simulink model "E13_implementation"  (R2017a)
settings: Solver=VariableStepAuto  StartTime=0.0  StopTime=50  RelTol=1e-3
InitFcn:
  | clear
  | E_param
undefined symbols (not defined in the file or in its folder): E_animation
settings Model: Creator=Mat Haskell  LastModifiedBy=Mat Haskell

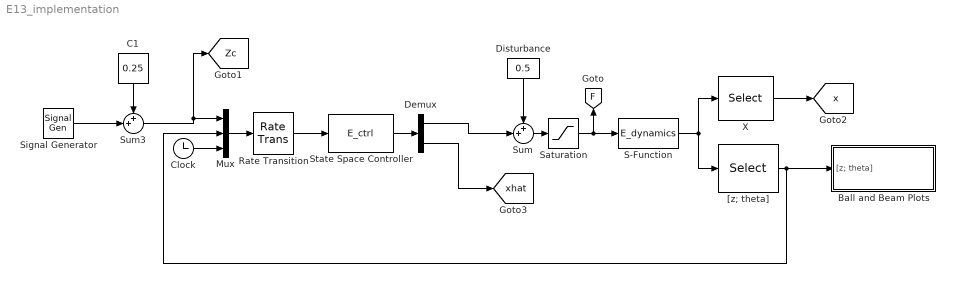
== system E13_implementation ==
  Ball and Beam Plots : Subsystem
  C1 : Constant  Value=0.25
  Clock : Clock
  Demux : Demux  Outputs=2
  Disturbance : Constant  Value=0.5
  Mux : Mux  Inputs=3
  Rate Transition : RateTransition  OutPortSampleTime=P.Ts
  S-Function : S-Function  FunctionName=E_dynamics  Parameters=P  SFunctionDeploymentMode=off  EnableBusSupport=off
  Saturation : Saturate  UpperLimit=15  LowerLimit=-15
  Signal Generator : SignalGenerator  WaveForm=square  Amplitude=.125  Frequency=.05
  State Space Controller : MATLABFcn  InitFcn=E_param  MATLABFcn=E_ctrl  OutputDimensions=5
  Sum : Sum  Inputs=++|
  Sum3 : Sum  Inputs=++|
  X : Selector  InputPortWidth=6  IndexOptions=Index vector (dialog)  Indices=[3 4 5 6]  OutputSizes=1
  "[z; theta]" : Selector  InputPortWidth=6  IndexOptions=Index vector (dialog)  Indices=[1 2]  OutputSizes=1
  tag scope: F=global, Zc=global, x=global, xhat=global
  wires:
  Sum3/1 -> [Zc], Mux/1
  Saturation/1 -> S-Function/1, [F]
  C1/1 -> Sum3/1
  Signal Generator/1 -> Sum3/2
  Sum/1 -> Saturation/1
  Disturbance/1 -> Sum/1
  Clock/1 -> Mux/3
  S-Function/1 -> X/1, "[z; theta]"/1
  X/1 -> [x]
  Demux/2 -> [xhat]
  "[z; theta]"/1 -> Mux/2, Ball and Beam Plots/1("[z; theta]")
  State Space Controller/1 -> Demux/1
  Demux/1 -> Sum/2
  Mux/1 -> Rate Transition/1
  Rate Transition/1 -> State Space Controller/1

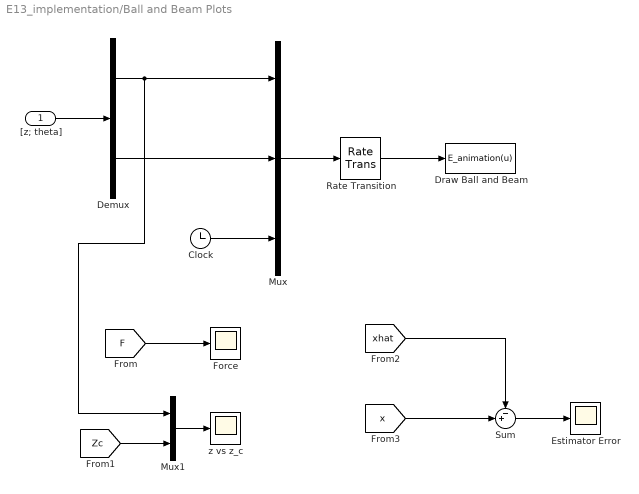
== system E13_implementation/Ball and Beam Plots ==
  "[z; theta]" : Inport
  Clock : Clock
  Demux : Demux  Outputs=2
  Draw Ball and Beam : MATLABFcn  MATLABFcn=E_animation(u)  OutputDimensions=0
  Estimator Error : Scope
  Force : Scope
  Mux : Mux  Inputs=3
  Mux1 : Mux  Inputs=2
  Rate Transition : RateTransition  OutPortSampleTime=P.t_plot
  Sum : Sum  Inputs=-+|
  z vs z_c : Scope
  wires:
  "[z; theta]"/1 -> Demux/1
  Rate Transition/1 -> Draw Ball and Beam/1
  Mux/1 -> Rate Transition/1
  Clock/1 -> Mux/3
  Demux/1 -> Mux1/1, Mux/1
  Demux/2 -> Mux/2
  [F] -> Force/1
  Mux1/1 -> z vs z_c/1
  [Zc] -> Mux1/2
  [xhat] -> Sum/1
  [x] -> Sum/2
  Sum/1 -> Estimator Error/1
